simulink subsystem "Loads"  (R2020a)
settings: Solver=VariableStepAuto  StartTime=0.0  StopTime=10.0  RelTol=1e-3
undefined symbols (not defined in the file): Angle, Speed, Torque, x28_000006_reduction
libraries: fl_lib x3, nesl_utility x3, sdl_lib x1
settings Model: Creator=khoi  LastModifiedBy=khoi

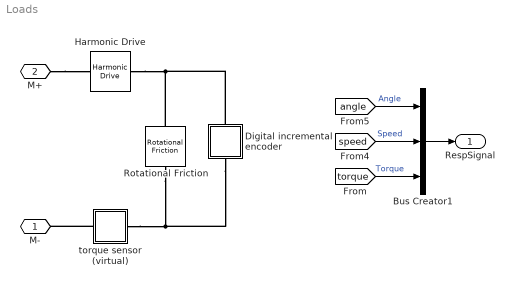
== system Loads ==
  Bus Creator1 : BusCreator  Inputs=Angle,Speed,Torque  OutDataTypeStr=Bus: RespSignal  NonVirtualBus=on
  Digital incremental encoder : Subsystem
      mask Display: disp('PV')
  Harmonic Drive : sdl_lib/Gears/Harmonic Drive  n_ellipse=x28_000006_reduction  n_circle=x28_000006_reduction+1  friction_model=1  T_noload=0.1 N*m  T_nom=5 N*m  efficiency_nom=.95  efficiency=.95  mu_visc=[0, 0] N*m/(rad/s)  w_thr=0.01 rad/s  pwr_thr=0.001 W  temperature_TLU=[280, 300, 320] K  load_TLU=[1, 5, 10] N*m  efficiency_TLU=[.95, .9, .85]  efficiency_TLU2=[.85, .8, .75; .95, .9, .85; .85, .8, .7]  thermal_mass=50 J/K  T_init=300 K
      settings: SourceProductBaseCode=LD  InternalSimscapePortConfiguration="{\"Bottom\":[],\"Left\":[{\"id\":\"B\",\"label\":\"B\",\"type\":\"foundation.mechanical.rotational.rotational\"}],\"Right\":[{\"id\":\"F\",\"label\":\"F\",\"type\":\"foundation.mechanical.rotational.rotational\"}],\"Top\":[]}"
  Rotational Friction : fl_lib/Mechanical/Rotational Elements/Rotational Friction  brkwy_trq=25 N*mm  brkwy_vel=0.1 rad/s  Col_trq=20 N*mm  visc_coef=0.001 N*m/(rad/s)  w_specify=off  w_priority=None  w=0 rad/s  w_nominal_specify=off  w_nominal_unit=rad/s  w_nominal_value=1  t_specify=off  t_priority=None  t=0 N*m  t_nominal_specify=off  t_nominal_unit=N*m  t_nominal_value=1
  torque sensor (virtual) : Subsystem
      mask Display: disp('T')
  M- : PMIOPort  Side=Left
  M+ : PMIOPort  Port=2  Side=Left
  RespSignal : Outport
  wires:
  [speed] -> Bus Creator1/2  "Speed"
  [angle] -> Bus Creator1/1  "Angle"
  Bus Creator1/1 -> RespSignal/1
  [torque] -> Bus Creator1/3  "Torque"
  connections:
  Rotational Friction/LConn1 -- Harmonic Drive/RConn1 -- Digital incremental encoder/LConn1
  torque sensor (virtual)/LConn1 -- Digital incremental encoder/RConn1 -- Rotational Friction/RConn1
  M+/RConn1 -- Harmonic Drive/LConn1
  torque sensor (virtual)/RConn1 -- M-/RConn1

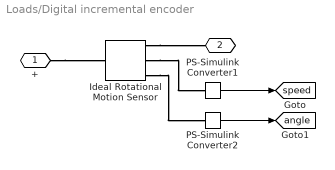
== system Loads/Digital incremental encoder ==
  Ideal Rotational Motion Sensor : fl_lib/Mechanical/Mechanical Sensors/Ideal Rotational Motion Sensor  wrap_angle=simscape.enum.onoff.off  offset=0 rad
  PS-Simulink Converter1 : nesl_utility/PS-Simulink Converter  PhysicalDomain=network_engine_domain  SubClassName=ps_output  LeftPortType=input  RightPortType=output  PseudoPeriodic=off  Frequencies=[]  Unit=rpm  AffineConversion=off
  PS-Simulink Converter2 : nesl_utility/PS-Simulink Converter  PhysicalDomain=network_engine_domain  SubClassName=ps_output  LeftPortType=input  RightPortType=output  PseudoPeriodic=off  Frequencies=[]  Unit=inherit  AffineConversion=off
  + : PMIOPort  Side=Left
  - : PMIOPort  Port=2  Side=Right
  tag scope: angle=global, speed=global
  wires:
  PS-Simulink Converter1/1 -> [speed]
  PS-Simulink Converter2/1 -> [angle]
  connections:
  Ideal Rotational Motion Sensor/RConn1 -- -/RConn1
  +/RConn1 -- Ideal Rotational Motion Sensor/LConn1
  Ideal Rotational Motion Sensor/RConn3 -- PS-Simulink Converter2/LConn1
  Ideal Rotational Motion Sensor/RConn2 -- PS-Simulink Converter1/LConn1

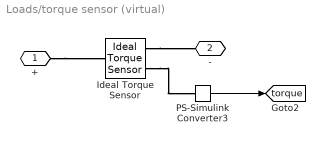
== system Loads/torque sensor (virtual) ==
  Ideal Torque Sensor : fl_lib/Mechanical/Mechanical Sensors/Ideal Torque Sensor
  PS-Simulink Converter3 : nesl_utility/PS-Simulink Converter  PhysicalDomain=network_engine_domain  SubClassName=ps_output  LeftPortType=input  RightPortType=output  PseudoPeriodic=off  Frequencies=[]  Unit=N*mm  AffineConversion=off
  + : PMIOPort  Side=Left
  - : PMIOPort  Port=2  Side=Right
  tag scope: torque=global
  wires:
  PS-Simulink Converter3/1 -> [torque]
  connections:
  Ideal Torque Sensor/RConn2 -- PS-Simulink Converter3/LConn1
  +/RConn1 -- Ideal Torque Sensor/LConn1
  Ideal Torque Sensor/RConn1 -- -/RConn1
